simulink model "double_3D_pend_Quat"  (R2023a)
settings: Solver=VariableStepAuto  StartTime=0.0  StopTime=5  MaxStep=1e-3  RelTol=1e-9  AbsTol=1e-9  EnableMultiTasking=on
InitFcn:
  | addpath MuscleForces\
  | addpath EquationsOfMotion\
  | data;
values from neighbouring files (symbols this model uses):
  activation = rand(6,1)    [data.m]    (also in initFunction.m = [0.1,0.5,0.1,0.1,0.1,0.1])
  force = rand(1,6)*500-250    [data.m]
  g = 9.81    [data.m]
  IL = [8.1667, 8.1667, 1.66667,0,0,0]    [data.m]
  IU = [8.1667, 8.1667, 1.66667,0,0,0]    [data.m]
  Ixx = 8.1667    [data.m]
  Iyy = 8.1667    [data.m]
  Izz = 1.66667    [data.m]
  l = 10    [data.m]
  l0m = [20,30,30,30,30,30]    [data.m]
  m = 5    [data.m]
  q1init = q1init/norm(q1init)    [data.m]    (also in initFunction.m)
undefined symbols (not defined in the file or in its folder): initialConditions, X, Y, Z
libraries: sm_lib x33, nesl_utility x15
settings Model: Creator=zoufi  LastModifiedBy=zoufi
settings SolverCC: AutoScaleAbsTol=off  AlgebraicLoopSolver=TrustRegion  MaxZcPerStep=1
settings DataIOCC: LimitDataPoints=on  MaxDataPoints=10000
settings OptimizationCC: ReuseModelBlockBuffer=off  LifeSpan=inf
settings DebuggingCC: UnconnectedInputMsg=warning  UnconnectedOutputMsg=warning  UnconnectedLineMsg=warning  AllowSymbolicDim=off  SubsystemReferenceDiagnosticForUnitTest=warning  SFUnexpectedBacktrackingDiag=warning  SFNoUnconditionalDefaultTransitionDiag=warning  SFExecutionAtInitializationDiag=none  ArithmeticOperatorsInVariantConditions=warning
settings ModelReferenceCC: EnableRefExpFcnMdlSchedulingChecks=on
settings SFSimCC: SimUseLocalCustomCode=off  CustomCodeUndefinedFunction=UseInterfaceOnly
settings RTWCC: RTWUseLocalCustomCode=off  DLArmComputeVersion=19.05
settings CodeAppCC: StateflowObjectComments=on
settings GRTTargetCC: TargetLangStandard=C89/C90 (ANSI)
settings ConfigComp: CovMetricSettings=dw  CovSaveCumulativeToWorkspaceVar=on  CovSaveSingleToWorkspaceVar=on  CovExternalEMLEnable=off  CovSFcnEnable=off
settings SimscapeCC: SimscapeLogType=all  SimscapeLogSimulationStatistics=on  SimscapeLogDataHistory=10000

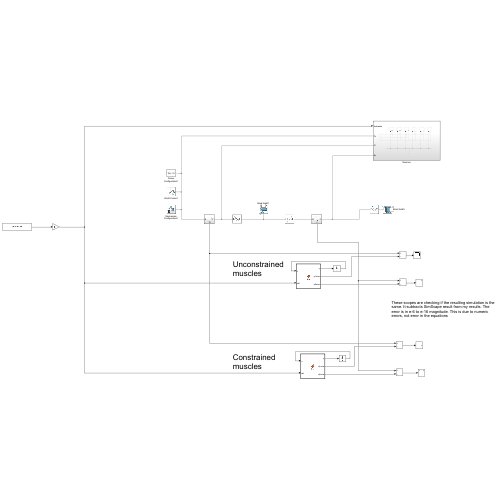
[thumbnail: Simulink's stored preview of the top-level diagram]
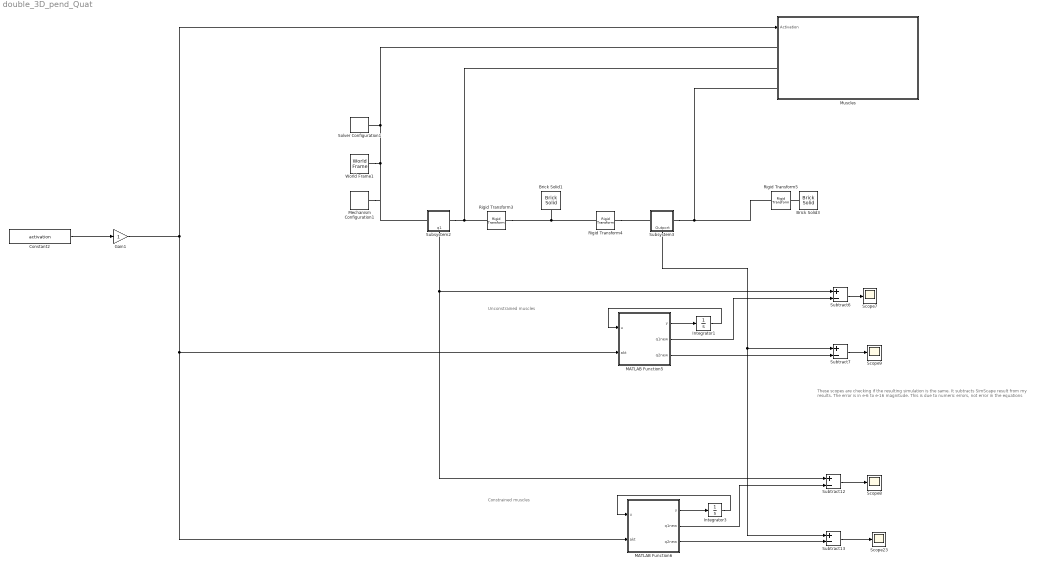
== system double_3D_pend_Quat ==
  note: These scopes are checking if the resulting simulation is the same. It subtracts SimScape result from my results. The error is in e-6 to e-16 magnitude. This is due to numeric errors, not error in the equations
  note: Unconstrained muscles
  note: Constrained muscles
  Brick Solid1 : sm_lib/Body Elements/Brick Solid  GraphicAmbientColor=[0.15 0.15 0.15 1.0]  BasedOnType=Density  BrickDimensions=[1 1 10]  BrickDimensionsUnits=m  CenterOfMass=[0 0 0]  CenterOfMassUnits=m  GraphicDiffuseColor=[0.5 0.5 0.5]  Density=1  DensityUnits=kg/m^3  DoExposeReferenceFrame=on  GraphicEmissiveColor=[0.0 0.0 0.0 1.0]  ExportEntireGeometry=off  SerializedFrames=<Frames><Frame><Id>Frame1</Id><Value><Name>nahore</Name><Origin><Source>GeometricFeature</Source><FeatureName>+z surface</FeatureName></Origin><PrimaryAxis><DefinedDirection>+Z</DefinedDirection><Source>ReferenceFrame</Source><SourceDirection>+Z</SourceDirection><FeatureName></FeatureName></PrimaryAxis><SecondaryAxis><DefinedDirection>+X</DefinedDirection><Source>ReferenceFrame</Source><SourceDirection>+X</SourceDirection><FeatureName></FeatureName></SecondaryAxis></Value></Frame><Frame><Id>Frame2</Id><Value><Name>dole</Name><Origin><Source>GeometricFeature</Source><FeatureName>-z surface</FeatureName></Origin><PrimaryAxis><DefinedDirection>+Z</DefinedDirection><Source>ReferenceFrame</Source><SourceDirection>+Z</SourceDirection><FeatureName></FeatureName></PrimaryAxis><SecondaryAxis><DefinedDirection>+X</DefinedDirection><Source>ReferenceFrame</Source><SourceDirection>+X</SourceDirection><FeatureName></FeatureName></SecondaryAxis></Value></Frame></Frames>  MarkerShape=Sphere  MarkerSize=10  GraphicType=FromGeometry  InertiaType=Custom  Mass=m  MassUnits=kg  MomentsOfInertia=IU(1:3)  MomentsOfInertiaUnits=kg*m^2  GraphicOpacity=1.0  ProductsOfInertia=IU(4:6)  ProductsOfInertiaUnits=kg*m^2  GraphicShininess=75  GraphicSpecularColor=[0.5 0.5 0.5 1.0]  GraphicVisPropType=SimpleVisualProperties
  Brick Solid3 : sm_lib/Body Elements/Brick Solid  GraphicAmbientColor=[0.15 0.15 0.15 1.0]  BasedOnType=Density  BrickDimensions=[1 1 10]  BrickDimensionsUnits=m  CenterOfMass=[0 0 0]  CenterOfMassUnits=m  GraphicDiffuseColor=[0.5 0.5 0.5]  Density=1  DensityUnits=kg/m^3  DoExposeReferenceFrame=on  GraphicEmissiveColor=[0.0 0.0 0.0 1.0]  ExportEntireGeometry=off  SerializedFrames=<Frames><Frame><Id>Frame1</Id><Value><Name>nahore</Name><Origin><Source>GeometricFeature</Source><FeatureName>+z surface</FeatureName></Origin><PrimaryAxis><DefinedDirection>+Z</DefinedDirection><Source>ReferenceFrame</Source><SourceDirection>+Z</SourceDirection><FeatureName></FeatureName></PrimaryAxis><SecondaryAxis><DefinedDirection>+X</DefinedDirection><Source>ReferenceFrame</Source><SourceDirection>+X</SourceDirection><FeatureName></FeatureName></SecondaryAxis></Value></Frame><Frame><Id>Frame2</Id><Value><Name>dole</Name><Origin><Source>GeometricFeature</Source><FeatureName>-z surface</FeatureName></Origin><PrimaryAxis><DefinedDirection>+Z</DefinedDirection><Source>ReferenceFrame</Source><SourceDirection>+Z</SourceDirection><FeatureName></FeatureName></PrimaryAxis><SecondaryAxis><DefinedDirection>+X</DefinedDirection><Source>ReferenceFrame</Source><SourceDirection>+X</SourceDirection><FeatureName></FeatureName></SecondaryAxis></Value></Frame></Frames>  MarkerShape=Sphere  MarkerSize=10  GraphicType=FromGeometry  InertiaType=Custom  Mass=m  MassUnits=kg  MomentsOfInertia=IL(1:3)  MomentsOfInertiaUnits=kg*m^2  GraphicOpacity=1.0  ProductsOfInertia=IL(4:6)  ProductsOfInertiaUnits=kg*m^2  GraphicShininess=75  GraphicSpecularColor=[0.5 0.5 0.5 1.0]  GraphicVisPropType=SimpleVisualProperties
  Constant2 : Constant  Value=activation
  Gain1 : Gain
  Integrator1 : Integrator  InitialCondition=[q1init';q2init';zeros(6,1)]
  Integrator3 : Integrator  InitialCondition=[q1init';q2init';zeros(6,1)]
  MATLAB Function5 : MATLAB Function  TreatAsAtomicUnit=on
  MATLAB Function6 : MATLAB Function  TreatAsAtomicUnit=on
  Mechanism Configuration1 : sm_lib/Utilities/Mechanism Configuration  UniformGravity=Constant  GravityVector=[0 0 -g]  GravityVectorUnits=m/s^2  LinearizationDelta=0.001  JointModeTransitionNonlinearIterations=2
  Muscles : Subsystem
  Rigid Transform3 : sm_lib/Frames and Transforms/Rigid Transform  TranslationMethod=Cartesian  TranslationStandardOffset=0  TranslationStandardOffsetUnits=m  TranslationStandardAxis=+Z  TranslationCartesianOffset=rigid1C  TranslationCartesianOffsetUnits=m  TranslationROffset=0  TranslationROffsetUnits=m  TranslationZOffset=0  TranslationZOffsetUnits=m  TranslationThetaOffset=0  TranslationThetaOffsetUnits=deg  RotationMethod=None  RotationAngleUnits=deg  RotationStandardAxis=+Z  RotationAngle=0.0  RotationArbitraryAxis=[0 0 1]  FollAlignAxisA=+X  BaseAlignAxisA=+Y  FollAlignAxisB=+Y  BaseAlignAxisB=+Z  RotationSequenceAxes=FollowerAxes  RotationSequence=XYX  RotationSequenceAngles=[0 0 0]  RotationSequenceAnglesUnits=deg  RotationMatrix=[1 0 0; 0 1 0; 0 0 1]  Quaternion=[1 0 0 0]
  Rigid Transform4 : sm_lib/Frames and Transforms/Rigid Transform  TranslationMethod=Cartesian  TranslationStandardOffset=0  TranslationStandardOffsetUnits=m  TranslationStandardAxis=+Z  TranslationCartesianOffset=rigid1P  TranslationCartesianOffsetUnits=m  TranslationROffset=0  TranslationROffsetUnits=m  TranslationZOffset=0  TranslationZOffsetUnits=m  TranslationThetaOffset=0  TranslationThetaOffsetUnits=deg  RotationMethod=None  RotationAngleUnits=deg  RotationStandardAxis=+Z  RotationAngle=0.0  RotationArbitraryAxis=[0 0 1]  FollAlignAxisA=+X  BaseAlignAxisA=+Y  FollAlignAxisB=+Y  BaseAlignAxisB=+Z  RotationSequenceAxes=FollowerAxes  RotationSequence=XYX  RotationSequenceAngles=[0 0 0]  RotationSequenceAnglesUnits=deg  RotationMatrix=[1 0 0; 0 1 0; 0 0 1]  Quaternion=[1 0 0 0]
  Rigid Transform5 : sm_lib/Frames and Transforms/Rigid Transform  TranslationMethod=Cartesian  TranslationStandardOffset=0  TranslationStandardOffsetUnits=m  TranslationStandardAxis=+Z  TranslationCartesianOffset=rigid2C  TranslationCartesianOffsetUnits=m  TranslationROffset=0  TranslationROffsetUnits=m  TranslationZOffset=0  TranslationZOffsetUnits=m  TranslationThetaOffset=0  TranslationThetaOffsetUnits=deg  RotationMethod=None  RotationAngleUnits=deg  RotationStandardAxis=+Z  RotationAngle=0.0  RotationArbitraryAxis=[0 0 1]  FollAlignAxisA=+X  BaseAlignAxisA=+Y  FollAlignAxisB=+Y  BaseAlignAxisB=+Z  RotationSequenceAxes=FollowerAxes  RotationSequence=XYX  RotationSequenceAngles=[0 0 0]  RotationSequenceAnglesUnits=deg  RotationMatrix=[1 0 0; 0 1 0; 0 0 1]  Quaternion=[1 0 0 0]
  Scope{7..9,23} (4 alike) : Scope
  Solver Configuration1 : nesl_utility/Solver Configuration  PhysicalDomain=network_engine_domain  SubClassName=solver  LeftPortType=input  RightPortType=generic  Tones=[]  Harmonics=[]  SimulateNoise=off  Profile=off  UseLocalSampling=off  EnableSwitchedLinearOptims=on  FrequencyDomain=off  UseCCode=off  RelTol=0.001  AbsTol=1e-06  MinStep=1e-09  ToWorkspace=off  RevertToSquareIcSolve=off  NumHomotopyIterations=100  PhasorMode=off  PhasorModeNumHarmonics=1  ConsistencySolver=NEWTON_XTOL_AFTER_FTOL  IndexReductionMethod=DerivativeReplacement  DoDC=off  ResidualTolerance=1e-09  ConsistencyTolSource=GLOBAL  ConsistencyAbsTol=0.001  ConsistencyRelTol=0.001  ConsistencyTolFactor=0.001  UseLocalSolver=off  LocalSolverChoice=NE_BACKWARD_EULER_ADVANCER  ResolveIndetEquations=on  FunctionEvalNumThread=1  LocalSolverSampleTime=0.001  DoFixedCost=off  MaxNonlinIter=3  MaxModeIter=2  ComputeImpulses=off  ImpulseIterations=2  LinearAlgebra=Sparse  LinearAlgebraNumThread=0  EquationFormulation=NE_TIME_EF  DelaysMemoryBudget=1024  AutomaticFiltering=on  FilteringTimeConstant=0.001  PartitionStorageMethod=AS_NEEDED  PartitionMemoryBudget=1024  PartitionMethod=FAST
  Subsystem2 : Subsystem
      settings: PortSchema="{\"entries\":[{\"content\":{\"sides\":[{\"content\":{\"connectorIds\":[\"LConn1\"]},\"type\":\"ConnectorPlacement.EquallySpacedRectSide\",\"uuid\":\"8abbfcc9-01b5-41c4-a283-6804113387f6\"},{\"content\":{\"connectorIds\":[\"RConn1\"],\"side\":\"RIGHT\"},\"type\":\"ConnectorPlacement.EquallySpacedRectSide\",\"uuid\":\"0343473e-44e7-4112-89d1-12c32e7e714a\"},{\"content\":{\"side\":\"TOP\"},\"type\":\"ConnectorPlacement.EquallySpacedRectSide\",\"uuid\":\"e3f3e934-10bc-4ce8-a108-92e62f8cce45\"},{\"content\":{\"connectorIds\":[\"Out1\"],\"side\":\"BOTTOM\"},\"type\":\"ConnectorPlacement.EquallySpacedRectSide\",\"uuid\":\"88cd244a-d5e6-4fc3-9229-ab44331ab4a2\"}]},\"type\":\"ConnectorPlacement.EquallySpacedConnector\",\"uuid\":\"3b604a58-c197-4bd4-84dd-7dfe8ba758a8\"}],\"packageUris\":[\"http://schema.mathworks.com/mf0/Connector/R2020b\"],\"version\":\"1.0\"}"
  Subsystem3 : Subsystem
      settings: PortSchema="{\"entries\":[{\"content\":{\"sides\":[{\"content\":{\"connectorIds\":[\"LConn1\"]},\"type\":\"ConnectorPlacement.EquallySpacedRectSide\",\"uuid\":\"a7767b74-3ef3-4a0a-9db8-74df01f0c76b\"},{\"content\":{\"connectorIds\":[\"RConn1\"],\"side\":\"RIGHT\"},\"type\":\"ConnectorPlacement.EquallySpacedRectSide\",\"uuid\":\"2f8f74c3-a8e5-4e43-9dec-7e8e5a722b87\"},{\"content\":{\"side\":\"TOP\"},\"type\":\"ConnectorPlacement.EquallySpacedRectSide\",\"uuid\":\"fe0d2add-2cc5-4054-90cf-1ce1d94f501e\"},{\"content\":{\"connectorIds\":[\"Out1\"],\"side\":\"BOTTOM\"},\"type\":\"ConnectorPlacement.EquallySpacedRectSide\",\"uuid\":\"7824871f-3418-47cc-a708-554774ed2fda\"}]},\"type\":\"ConnectorPlacement.EquallySpacedConnector\",\"uuid\":\"6ea328c6-953a-4acc-92cd-0e7443fdf9ea\"}],\"packageUris\":[\"http://schema.mathworks.com/mf0/Connector/R2020b\"],\"version\":\"1.0\"}"
  Subtract{6..7,12..13} (4 alike) : Sum  Inputs=+-
  World Frame1 : sm_lib/Frames and Transforms/World Frame
  wires:
  Constant2/1 -> Gain1/1
  MATLAB Function5/1(y) -> Integrator1/1
  Integrator1/1 -> MATLAB Function5/1(u)
  MATLAB Function5/2(q1new) -> Subtract6/2
  Subtract6/1 -> Scope7/1
  MATLAB Function5/3(q2new) -> Subtract7/2
  Subtract7/1 -> Scope9/1
  Subsystem3/1(Outport) -> Subtract13/1, Subtract7/1
  Subtract13/1 -> Scope23/1
  MATLAB Function6/3(q2new) -> Subtract13/2
  Subtract12/1 -> Scope8/1
  MATLAB Function6/2(q1new) -> Subtract12/2
  Subsystem2/1(q1) -> Subtract12/1, Subtract6/1
  Integrator3/1 -> MATLAB Function6/1(u)
  MATLAB Function6/1(y) -> Integrator3/1
  Gain1/1 -> Muscles/1(Activation), MATLAB Function6/2(akt), MATLAB Function5/2(akt)
  connections:
  World Frame1/RConn1 -- Muscles/LConn1 -- Solver Configuration1/RConn1 -- Subsystem2/LConn1 -- Mechanism Configuration1/RConn1
  Subsystem2/RConn1 -- Muscles/LConn2 -- Rigid Transform3/RConn1
  Rigid Transform3/LConn1 -- Rigid Transform4/LConn1 -- Brick Solid1/RConn1
  Brick Solid3/RConn1 -- Rigid Transform5/LConn1
  Subsystem3/RConn1 -- Muscles/LConn3 -- Rigid Transform5/RConn1
  Rigid Transform4/RConn1 -- Subsystem3/LConn1

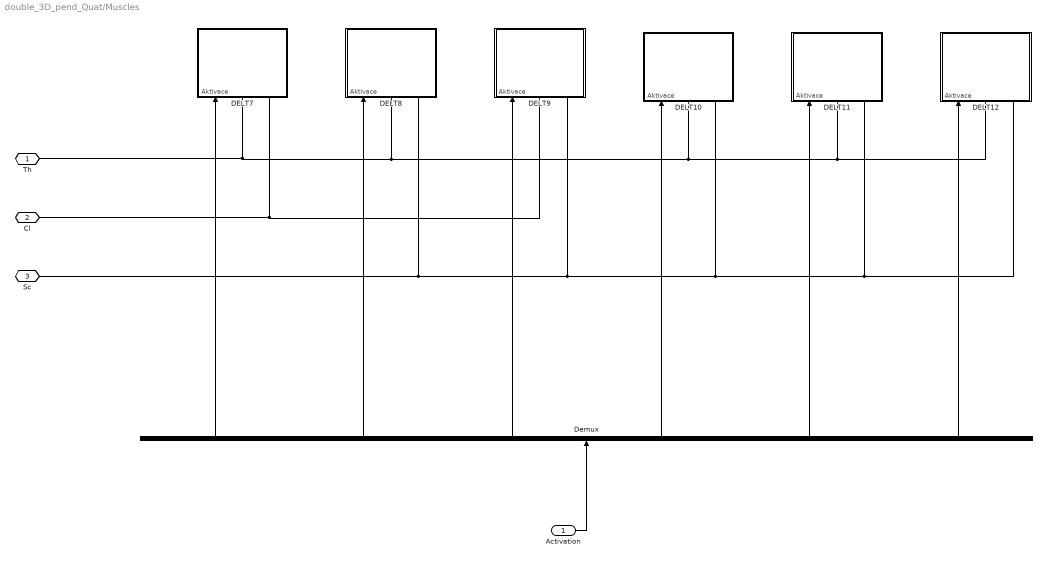
== system double_3D_pend_Quat/Muscles ==
  Activation : Inport
  DELT10 : Subsystem
  DELT11 : Subsystem
  DELT12 : Subsystem
  DELT7 : Subsystem
  DELT8 : Subsystem
  DELT9 : Subsystem
  Demux : Demux  Outputs=6
  Th : PMIOPort  Side=Left
  Cl : PMIOPort  Port=2  Side=Left
  Sc : PMIOPort  Port=3  Side=Left
  wires:
  Demux/1 -> DELT7/1(Aktivace)
  Demux/2 -> DELT8/1(Aktivace)
  Demux/3 -> DELT9/1(Aktivace)
  Demux/4 -> DELT10/1(Aktivace)
  Demux/5 -> DELT11/1(Aktivace)
  Demux/6 -> DELT12/1(Aktivace)
  Activation/1 -> Demux/1
  connections:
  DELT7/LConn1 -- DELT12/LConn1 -- DELT11/LConn1 -- DELT10/LConn1 -- DELT8/LConn1 -- Th/RConn1
  DELT7/LConn2 -- DELT9/LConn1 -- Cl/RConn1
  DELT8/LConn2 -- DELT12/LConn2 -- DELT11/LConn2 -- DELT10/LConn2 -- DELT9/LConn2 -- Sc/RConn1

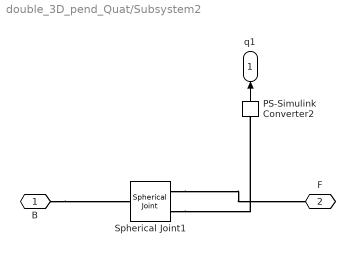
== system double_3D_pend_Quat/Subsystem2 ==
  PS-Simulink Converter2 : nesl_utility/PS-Simulink Converter  PhysicalDomain=network_engine_domain  SubClassName=ps_output  LeftPortType=input  RightPortType=output  PseudoPeriodic=off  Frequencies=[]  VectorFormat=inherit  Unit=inherit  AffineConversion=off
  Spherical Joint1 : sm_lib/Joints/Spherical Joint  JointMode=Normal  SenseConstraintForce=off  SenseConstraintForceX=off  SenseConstraintForceY=off  SenseConstraintForceZ=off  SenseConstraintTorque=off  SenseConstraintTorqueX=off  SenseConstraintTorqueY=off  SenseConstraintTorqueZ=off  SenseTotalForce=off  SenseTotalForceX=off  SenseTotalForceY=off  SenseTotalForceZ=off  SenseTotalTorque=off  SenseTotalTorqueX=off  SenseTotalTorqueY=off  SenseTotalTorqueZ=off  CompositeWrenchDir=BaseOnFollower  CompositeWrenchFrame=BaseFrame  EqPosRotationMethod=None  EqPosRotationAngleUnits=deg  EqPosRotationStandardAxis=+Z  EqPosRotationAngle=0.0  EqPosRotationArbitraryAxis=[0 0 1]  EqPosFollAlignAxisA=+X  EqPosBaseAlignAxisA=+Y  EqPosFollAlignAxisB=+Y  EqPosBaseAlignAxisB=+Z  EqPosRotationSequenceAxes=FollowerAxes  EqPosRotationSequence=XYX  EqPosRotationSequenceAngles=[0 0 0]  EqPosRotationSequenceAnglesUnits=deg  EqPosRotationMatrix=[1 0 0; 0 1 0; 0 0 1]  EqPosQuaternion=[1 0 0 0]  SpringStiffness=0  SpringStiffnessUnits=N*m/deg  DampingCoefficient=c  DampingCoefficientUnits=N*m/(rad/s)  ActuateTorqueX=off  ActuateTorqueY=off  ActuateTorqueZ=off  ActuateTorque=off  TorqueActuationMode=InputTorque  MotionActuationMode=ComputedMotion  ActuationFrame=FollowerFrame  SensePosition=on  SenseVelocityX=off  SenseVelocityY=off  SenseVelocityZ=off  SenseVelocity=off  SenseAccelerationX=off  SenseAccelerationY=off  SenseAccelerationZ=off  SenseAcceleration=off  SenseTorqueX=off  SenseTorqueY=off  SenseTorqueZ=off  SenseTorqueForce=off  SenseLowerLimitTorqueMag=off  SenseUpperLimitTorqueMag=off  SensingFrame=BaseFrame  LowerLimitSpecify=off  LowerLimitBound=15  LowerLimitBoundUnits=deg  LowerLimitStiffness=1e4  LowerLimitStiffnessUnits=N*m/deg  LowerLimitDamping=10  LowerLimitDampingUnits=N*m/(deg/s)  LowerLimitTransitionRegionWidth=0.1  LowerLimitTransitionRegionWidthUnits=deg  UpperLimitSpecify=off  UpperLimitBound=45  UpperLimitBoundUnits=deg  UpperLimitStiffness=1e4  UpperLimitStiffnessUnits=N*m/deg  UpperLimitDamping=10  UpperLimitDampingUnits=N*m/(deg/s)  UpperLimitTransitionRegionWidth=0.1  UpperLimitTransitionRegionWidthUnits=deg  PositionTargetRotationMethod=Quaternion  PositionTargetRotationAngleUnits=deg  PositionTargetRotationStandardAxis=+Z  PositionTargetRotationAngle=0.0  PositionTargetRotationArbitraryAxis=[0 0 1]  PositionTargetFollAlignAxisA=+X  PositionTargetBaseAlignAxisA=+Y  PositionTargetFollAlignAxisB=+Y  PositionTargetBaseAlignAxisB=+Z  PositionTargetRotationSequenceAxes=FollowerAxes  PositionTargetRotationSequence=XYZ  PositionTargetRotationSequenceAngles=initialConditions(1:3)  PositionTargetRotationSequenceAnglesUnits=rad  PositionTargetRotationMatrix=[1 0 0; 0 1 0; 0 0 1]  PositionTargetQuaternion=q1init  PositionTargetSpecify=on  PositionTargetPriority=High  VelocityTargetValue=[0 0 0]  VelocityTargetValueUnits=deg/s  VelocityTargetSpecify=off  VelocityTargetPriority=High  VelocityTargetInFollowerFrame=on
  B : PMIOPort  Side=Left
  F : PMIOPort  Port=2  Side=Right
  q1 : Outport
  wires:
  PS-Simulink Converter2/1 -> q1/1
  connections:
  Spherical Joint1/RConn2 -- PS-Simulink Converter2/LConn1
  Spherical Joint1/RConn1 -- F/RConn1
  B/RConn1 -- Spherical Joint1/LConn1

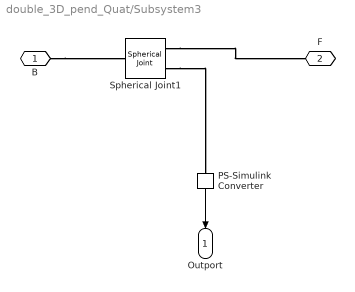
== system double_3D_pend_Quat/Subsystem3 ==
  PS-Simulink Converter : nesl_utility/PS-Simulink Converter  PhysicalDomain=network_engine_domain  SubClassName=ps_output  LeftPortType=input  RightPortType=output  PseudoPeriodic=off  Frequencies=[]  VectorFormat=inherit  Unit=inherit  AffineConversion=off
  Spherical Joint1 : sm_lib/Joints/Spherical Joint  JointMode=Normal  SenseConstraintForce=off  SenseConstraintForceX=off  SenseConstraintForceY=off  SenseConstraintForceZ=off  SenseConstraintTorque=off  SenseConstraintTorqueX=off  SenseConstraintTorqueY=off  SenseConstraintTorqueZ=off  SenseTotalForce=off  SenseTotalForceX=off  SenseTotalForceY=off  SenseTotalForceZ=off  SenseTotalTorque=off  SenseTotalTorqueX=off  SenseTotalTorqueY=off  SenseTotalTorqueZ=off  CompositeWrenchDir=FollowerOnBase  CompositeWrenchFrame=BaseFrame  EqPosRotationMethod=None  EqPosRotationAngleUnits=deg  EqPosRotationStandardAxis=+Z  EqPosRotationAngle=0.0  EqPosRotationArbitraryAxis=[0 0 1]  EqPosFollAlignAxisA=+X  EqPosBaseAlignAxisA=+Y  EqPosFollAlignAxisB=+Y  EqPosBaseAlignAxisB=+Z  EqPosRotationSequenceAxes=FollowerAxes  EqPosRotationSequence=XYX  EqPosRotationSequenceAngles=[0 0 0]  EqPosRotationSequenceAnglesUnits=deg  EqPosRotationMatrix=[1 0 0; 0 1 0; 0 0 1]  EqPosQuaternion=[1 0 0 0]  SpringStiffness=0  SpringStiffnessUnits=N*m/deg  DampingCoefficient=c  DampingCoefficientUnits=N*m/(rad/s)  ActuateTorqueX=off  ActuateTorqueY=off  ActuateTorqueZ=off  ActuateTorque=off  TorqueActuationMode=InputTorque  MotionActuationMode=ComputedMotion  ActuationFrame=FollowerFrame  SensePosition=on  SenseVelocityX=off  SenseVelocityY=off  SenseVelocityZ=off  SenseVelocity=off  SenseAccelerationX=off  SenseAccelerationY=off  SenseAccelerationZ=off  SenseAcceleration=off  SenseTorqueX=off  SenseTorqueY=off  SenseTorqueZ=off  SenseTorqueForce=off  SenseLowerLimitTorqueMag=off  SenseUpperLimitTorqueMag=off  SensingFrame=BaseFrame  LowerLimitSpecify=off  LowerLimitBound=15  LowerLimitBoundUnits=deg  LowerLimitStiffness=1e4  LowerLimitStiffnessUnits=N*m/deg  LowerLimitDamping=10  LowerLimitDampingUnits=N*m/(deg/s)  LowerLimitTransitionRegionWidth=0.1  LowerLimitTransitionRegionWidthUnits=deg  UpperLimitSpecify=off  UpperLimitBound=45  UpperLimitBoundUnits=deg  UpperLimitStiffness=1e4  UpperLimitStiffnessUnits=N*m/deg  UpperLimitDamping=10  UpperLimitDampingUnits=N*m/(deg/s)  UpperLimitTransitionRegionWidth=0.1  UpperLimitTransitionRegionWidthUnits=deg  PositionTargetRotationMethod=Quaternion  PositionTargetRotationAngleUnits=deg  PositionTargetRotationStandardAxis=+Z  PositionTargetRotationAngle=0.0  PositionTargetRotationArbitraryAxis=[0 0 1]  PositionTargetFollAlignAxisA=+X  PositionTargetBaseAlignAxisA=+Y  PositionTargetFollAlignAxisB=+Y  PositionTargetBaseAlignAxisB=+Z  PositionTargetRotationSequenceAxes=FollowerAxes  PositionTargetRotationSequence=XYZ  PositionTargetRotationSequenceAngles=initialConditions(4:6)  PositionTargetRotationSequenceAnglesUnits=rad  PositionTargetRotationMatrix=[1 0 0; 0 1 0; 0 0 1]  PositionTargetQuaternion=q2init  PositionTargetSpecify=on  PositionTargetPriority=High  VelocityTargetValue=[0 0 0]  VelocityTargetValueUnits=deg/s  VelocityTargetSpecify=off  VelocityTargetPriority=High  VelocityTargetInFollowerFrame=on
  B : PMIOPort  Side=Left
  F : PMIOPort  Port=2  Side=Right
  Outport : Outport
  wires:
  PS-Simulink Converter/1 -> Outport/1
  connections:
  B/RConn1 -- Spherical Joint1/LConn1
  Spherical Joint1/RConn1 -- F/RConn1
  Spherical Joint1/RConn2 -- PS-Simulink Converter/LConn1

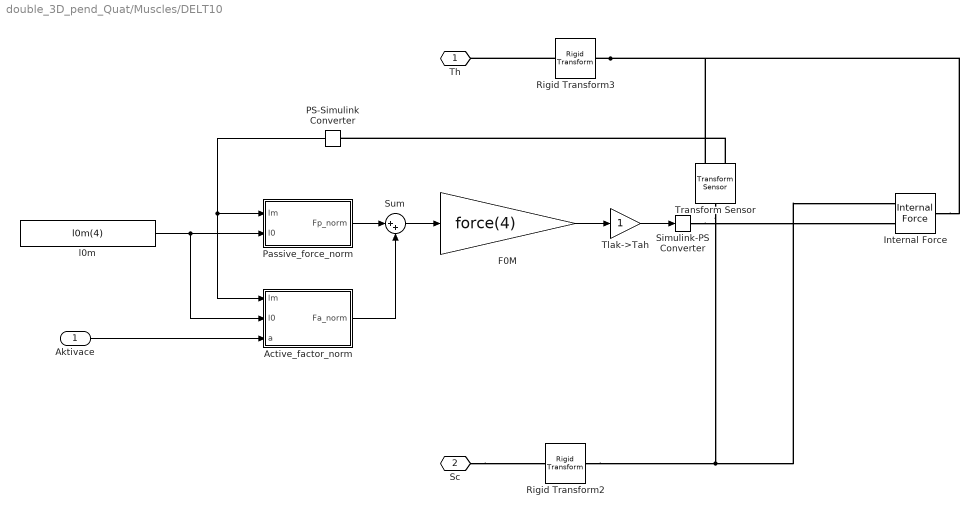
== system double_3D_pend_Quat/Muscles/DELT10 ==
  Aktivace : Inport
  Active_factor_norm : MATLAB Function  TreatAsAtomicUnit=on
  F0M : Gain  Gain=force(4)
  Internal Force : sm_lib/Forces and Torques/Internal Force
  PS-Simulink Converter : nesl_utility/PS-Simulink Converter  PhysicalDomain=network_engine_domain  SubClassName=ps_output  LeftPortType=input  RightPortType=output  PseudoPeriodic=off  Frequencies=[]  VectorFormat=inherit  Unit=inherit  AffineConversion=off
  Passive_force_norm : MATLAB Function  TreatAsAtomicUnit=on
  Rigid Transform2 : sm_lib/Frames and Transforms/Rigid Transform  TranslationMethod=Cartesian  TranslationStandardOffset=0  TranslationStandardOffsetUnits=m  TranslationStandardAxis=+Z  TranslationCartesianOffset=[2,-2,5]  TranslationCartesianOffsetUnits=m  TranslationROffset=0  TranslationROffsetUnits=m  TranslationZOffset=0  TranslationZOffsetUnits=m  TranslationThetaOffset=0  TranslationThetaOffsetUnits=deg  RotationMethod=None  RotationAngleUnits=deg  RotationStandardAxis=+Z  RotationAngle=0.0  RotationArbitraryAxis=[0 0 1]  FollAlignAxisA=+X  BaseAlignAxisA=+Y  FollAlignAxisB=+Y  BaseAlignAxisB=+Z  RotationSequenceAxes=FollowerAxes  RotationSequence=XYX  RotationSequenceAngles=[0 0 0]  RotationSequenceAnglesUnits=deg  RotationMatrix=[1 0 0; 0 1 0; 0 0 1]  Quaternion=[1 0 0 0]
  Rigid Transform3 : sm_lib/Frames and Transforms/Rigid Transform  TranslationMethod=Cartesian  TranslationStandardOffset=0  TranslationStandardOffsetUnits=m  TranslationStandardAxis=+Z  TranslationCartesianOffset=[-6, -6, 0]  TranslationCartesianOffsetUnits=m  TranslationROffset=0  TranslationROffsetUnits=m  TranslationZOffset=0  TranslationZOffsetUnits=m  TranslationThetaOffset=0  TranslationThetaOffsetUnits=deg  RotationMethod=None  RotationAngleUnits=deg  RotationStandardAxis=+Z  RotationAngle=0.0  RotationArbitraryAxis=[0 0 1]  FollAlignAxisA=+X  BaseAlignAxisA=+Y  FollAlignAxisB=+Y  BaseAlignAxisB=+Z  RotationSequenceAxes=FollowerAxes  RotationSequence=XYX  RotationSequenceAngles=[0 0 0]  RotationSequenceAnglesUnits=deg  RotationMatrix=[1 0 0; 0 1 0; 0 0 1]  Quaternion=[1 0 0 0]
  Simulink-PS Converter : nesl_utility/Simulink-PS Converter  PhysicalDomain=network_engine_domain  SubClassName=ps_input  LeftPortType=input  RightPortType=output  PseudoPeriodic=off  Frequencies=[]  NoiseDistribution=none  NoiseParameters=[]  Unit=1  AffineConversion=off  FilteringAndDerivatives=provide  SimscapeFilterOrder=1  InputFilterTimeConstant=0.001  UdotUserProvided=0
  Sum : Sum  Inputs=|++
  Tlak->Tah : Gain
  Transform Sensor : sm_lib/Frames and Transforms/Transform Sensor  MeasurementFrame=World  RotationSequence=XYX  SenseAngle=off  SenseAxis=off  SenseQ=off  SenseR=off  SenseRotationSequence=off  SenseOmegaX=off  SenseOmegaY=off  SenseOmegaZ=off  SenseQDot=off  SenseRDot=off  SenseRotationSequenceDot=off  SenseAlphaX=off  SenseAlphaY=off  SenseAlphaZ=off  SenseQDDot=off  SenseRDDot=off  SenseX=off  SenseY=off  SenseZ=off  SenseRad=off  SenseAzim=off  SenseDist=on  SenseInc=off  SenseXDot=off  SenseYDot=off  SenseZDot=off  SenseRadDot=off  SenseAzimDot=off  SenseDistDot=off  SenseIncDot=off  SenseXDDot=off  SenseYDDot=off  SenseZDDot=off  SenseRadDDot=off  SenseAzimDDot=off  SenseDistDDot=off  SenseIncDDot=off
  l0m : Constant  Value=l0m(4)
  Th : PMIOPort  Side=Left
  Sc : PMIOPort  Port=2  Side=Left
  wires:
  Aktivace/1 -> Active_factor_norm/3(a)
  l0m/1 -> Passive_force_norm/2(l0), Active_factor_norm/2(l0)
  PS-Simulink Converter/1 -> Passive_force_norm/1(lm), Active_factor_norm/1(lm)
  Tlak->Tah/1 -> Simulink-PS Converter/1
  Active_factor_norm/1(Fa_norm) -> Sum/2
  Passive_force_norm/1(Fp_norm) -> Sum/1
  F0M/1 -> Tlak->Tah/1
  Sum/1 -> F0M/1
  connections:
  Transform Sensor/RConn2 -- PS-Simulink Converter/LConn1
  Simulink-PS Converter/RConn1 -- Internal Force/LConn2
  Rigid Transform3/RConn1 -- Transform Sensor/RConn1 -- Internal Force/RConn1
  Transform Sensor/LConn1 -- Rigid Transform2/RConn1 -- Internal Force/LConn1
  Rigid Transform3/LConn1 -- Th/RConn1
  Sc/RConn1 -- Rigid Transform2/LConn1

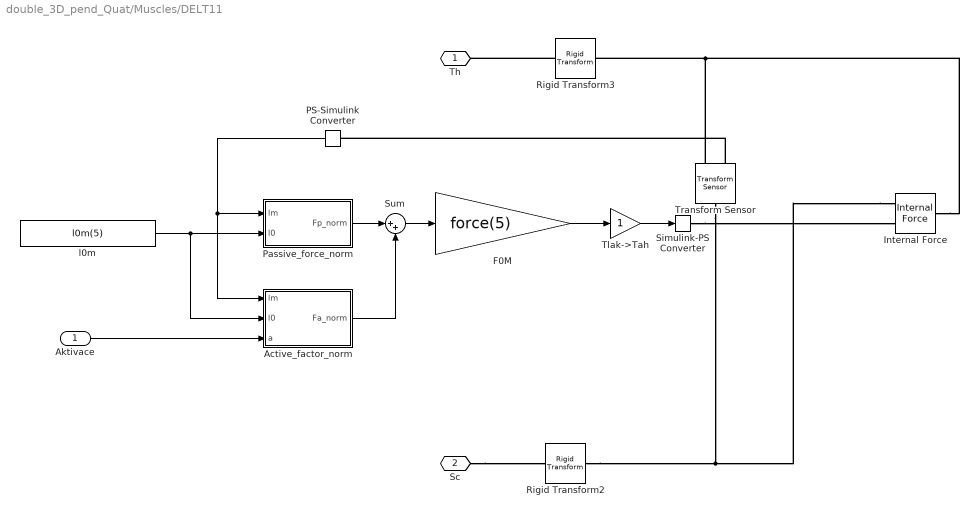
== system double_3D_pend_Quat/Muscles/DELT11 ==
  Aktivace : Inport
  Active_factor_norm : MATLAB Function  TreatAsAtomicUnit=on
  F0M : Gain  Gain=force(5)
  Internal Force : sm_lib/Forces and Torques/Internal Force
  PS-Simulink Converter : nesl_utility/PS-Simulink Converter  PhysicalDomain=network_engine_domain  SubClassName=ps_output  LeftPortType=input  RightPortType=output  PseudoPeriodic=off  Frequencies=[]  VectorFormat=inherit  Unit=inherit  AffineConversion=off
  Passive_force_norm : MATLAB Function  TreatAsAtomicUnit=on
  Rigid Transform2 : sm_lib/Frames and Transforms/Rigid Transform  TranslationMethod=Cartesian  TranslationStandardOffset=0  TranslationStandardOffsetUnits=m  TranslationStandardAxis=+Z  TranslationCartesianOffset=[-3,-3,0]  TranslationCartesianOffsetUnits=m  TranslationROffset=0  TranslationROffsetUnits=m  TranslationZOffset=0  TranslationZOffsetUnits=m  TranslationThetaOffset=0  TranslationThetaOffsetUnits=deg  RotationMethod=None  RotationAngleUnits=deg  RotationStandardAxis=+Z  RotationAngle=0.0  RotationArbitraryAxis=[0 0 1]  FollAlignAxisA=+X  BaseAlignAxisA=+Y  FollAlignAxisB=+Y  BaseAlignAxisB=+Z  RotationSequenceAxes=FollowerAxes  RotationSequence=XYX  RotationSequenceAngles=[0 0 0]  RotationSequenceAnglesUnits=deg  RotationMatrix=[1 0 0; 0 1 0; 0 0 1]  Quaternion=[1 0 0 0]
  Rigid Transform3 : sm_lib/Frames and Transforms/Rigid Transform  TranslationMethod=Cartesian  TranslationStandardOffset=0  TranslationStandardOffsetUnits=m  TranslationStandardAxis=+Z  TranslationCartesianOffset=[-7, 5, 0]  TranslationCartesianOffsetUnits=m  TranslationROffset=0  TranslationROffsetUnits=m  TranslationZOffset=0  TranslationZOffsetUnits=m  TranslationThetaOffset=0  TranslationThetaOffsetUnits=deg  RotationMethod=None  RotationAngleUnits=deg  RotationStandardAxis=+Z  RotationAngle=0.0  RotationArbitraryAxis=[0 0 1]  FollAlignAxisA=+X  BaseAlignAxisA=+Y  FollAlignAxisB=+Y  BaseAlignAxisB=+Z  RotationSequenceAxes=FollowerAxes  RotationSequence=XYX  RotationSequenceAngles=[0 0 0]  RotationSequenceAnglesUnits=deg  RotationMatrix=[1 0 0; 0 1 0; 0 0 1]  Quaternion=[1 0 0 0]
  Simulink-PS Converter : nesl_utility/Simulink-PS Converter  PhysicalDomain=network_engine_domain  SubClassName=ps_input  LeftPortType=input  RightPortType=output  PseudoPeriodic=off  Frequencies=[]  NoiseDistribution=none  NoiseParameters=[]  Unit=1  AffineConversion=off  FilteringAndDerivatives=provide  SimscapeFilterOrder=1  InputFilterTimeConstant=0.001  UdotUserProvided=0
  Sum : Sum  Inputs=|++
  Tlak->Tah : Gain
  Transform Sensor : sm_lib/Frames and Transforms/Transform Sensor  MeasurementFrame=World  RotationSequence=XYX  SenseAngle=off  SenseAxis=off  SenseQ=off  SenseR=off  SenseRotationSequence=off  SenseOmegaX=off  SenseOmegaY=off  SenseOmegaZ=off  SenseQDot=off  SenseRDot=off  SenseRotationSequenceDot=off  SenseAlphaX=off  SenseAlphaY=off  SenseAlphaZ=off  SenseQDDot=off  SenseRDDot=off  SenseX=off  SenseY=off  SenseZ=off  SenseRad=off  SenseAzim=off  SenseDist=on  SenseInc=off  SenseXDot=off  SenseYDot=off  SenseZDot=off  SenseRadDot=off  SenseAzimDot=off  SenseDistDot=off  SenseIncDot=off  SenseXDDot=off  SenseYDDot=off  SenseZDDot=off  SenseRadDDot=off  SenseAzimDDot=off  SenseDistDDot=off  SenseIncDDot=off
  l0m : Constant  Value=l0m(5)
  Th : PMIOPort  Side=Left
  Sc : PMIOPort  Port=2  Side=Left
  wires:
  Sum/1 -> F0M/1
  F0M/1 -> Tlak->Tah/1
  Passive_force_norm/1(Fp_norm) -> Sum/1
  Active_factor_norm/1(Fa_norm) -> Sum/2
  Tlak->Tah/1 -> Simulink-PS Converter/1
  PS-Simulink Converter/1 -> Active_factor_norm/1(lm), Passive_force_norm/1(lm)
  l0m/1 -> Active_factor_norm/2(l0), Passive_force_norm/2(l0)
  Aktivace/1 -> Active_factor_norm/3(a)
  connections:
  Sc/RConn1 -- Rigid Transform2/LConn1
  Rigid Transform3/LConn1 -- Th/RConn1
  Internal Force/LConn1 -- Rigid Transform2/RConn1 -- Transform Sensor/LConn1
  Internal Force/RConn1 -- Transform Sensor/RConn1 -- Rigid Transform3/RConn1
  Simulink-PS Converter/RConn1 -- Internal Force/LConn2
  Transform Sensor/RConn2 -- PS-Simulink Converter/LConn1

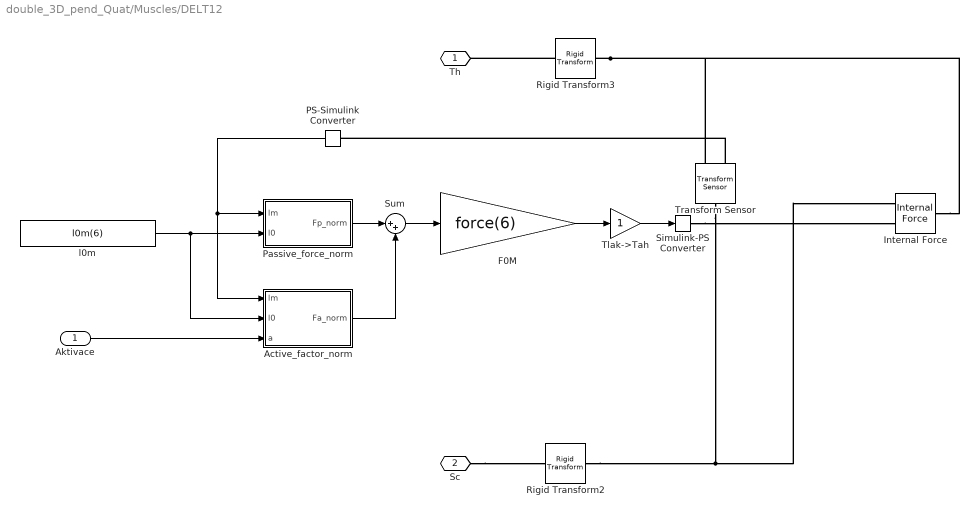
== system double_3D_pend_Quat/Muscles/DELT12 ==
  Aktivace : Inport
  Active_factor_norm : MATLAB Function  TreatAsAtomicUnit=on
  F0M : Gain  Gain=force(6)
  Internal Force : sm_lib/Forces and Torques/Internal Force
  PS-Simulink Converter : nesl_utility/PS-Simulink Converter  PhysicalDomain=network_engine_domain  SubClassName=ps_output  LeftPortType=input  RightPortType=output  PseudoPeriodic=off  Frequencies=[]  VectorFormat=inherit  Unit=inherit  AffineConversion=off
  Passive_force_norm : MATLAB Function  TreatAsAtomicUnit=on
  Rigid Transform2 : sm_lib/Frames and Transforms/Rigid Transform  TranslationMethod=Cartesian  TranslationStandardOffset=0  TranslationStandardOffsetUnits=m  TranslationStandardAxis=+Z  TranslationCartesianOffset=[-4,4,-4]  TranslationCartesianOffsetUnits=m  TranslationROffset=0  TranslationROffsetUnits=m  TranslationZOffset=0  TranslationZOffsetUnits=m  TranslationThetaOffset=0  TranslationThetaOffsetUnits=deg  RotationMethod=None  RotationAngleUnits=deg  RotationStandardAxis=+Z  RotationAngle=0.0  RotationArbitraryAxis=[0 0 1]  FollAlignAxisA=+X  BaseAlignAxisA=+Y  FollAlignAxisB=+Y  BaseAlignAxisB=+Z  RotationSequenceAxes=FollowerAxes  RotationSequence=XYX  RotationSequenceAngles=[0 0 0]  RotationSequenceAnglesUnits=deg  RotationMatrix=[1 0 0; 0 1 0; 0 0 1]  Quaternion=[1 0 0 0]
  Rigid Transform3 : sm_lib/Frames and Transforms/Rigid Transform  TranslationMethod=Cartesian  TranslationStandardOffset=0  TranslationStandardOffsetUnits=m  TranslationStandardAxis=+Z  TranslationCartesianOffset=[8, -4, 0]  TranslationCartesianOffsetUnits=m  TranslationROffset=0  TranslationROffsetUnits=m  TranslationZOffset=0  TranslationZOffsetUnits=m  TranslationThetaOffset=0  TranslationThetaOffsetUnits=deg  RotationMethod=None  RotationAngleUnits=deg  RotationStandardAxis=+Z  RotationAngle=0.0  RotationArbitraryAxis=[0 0 1]  FollAlignAxisA=+X  BaseAlignAxisA=+Y  FollAlignAxisB=+Y  BaseAlignAxisB=+Z  RotationSequenceAxes=FollowerAxes  RotationSequence=XYX  RotationSequenceAngles=[0 0 0]  RotationSequenceAnglesUnits=deg  RotationMatrix=[1 0 0; 0 1 0; 0 0 1]  Quaternion=[1 0 0 0]
  Simulink-PS Converter : nesl_utility/Simulink-PS Converter  PhysicalDomain=network_engine_domain  SubClassName=ps_input  LeftPortType=input  RightPortType=output  PseudoPeriodic=off  Frequencies=[]  NoiseDistribution=none  NoiseParameters=[]  Unit=1  AffineConversion=off  FilteringAndDerivatives=provide  SimscapeFilterOrder=1  InputFilterTimeConstant=0.001  UdotUserProvided=0
  Sum : Sum  Inputs=|++
  Tlak->Tah : Gain
  Transform Sensor : sm_lib/Frames and Transforms/Transform Sensor  MeasurementFrame=World  RotationSequence=XYX  SenseAngle=off  SenseAxis=off  SenseQ=off  SenseR=off  SenseRotationSequence=off  SenseOmegaX=off  SenseOmegaY=off  SenseOmegaZ=off  SenseQDot=off  SenseRDot=off  SenseRotationSequenceDot=off  SenseAlphaX=off  SenseAlphaY=off  SenseAlphaZ=off  SenseQDDot=off  SenseRDDot=off  SenseX=off  SenseY=off  SenseZ=off  SenseRad=off  SenseAzim=off  SenseDist=on  SenseInc=off  SenseXDot=off  SenseYDot=off  SenseZDot=off  SenseRadDot=off  SenseAzimDot=off  SenseDistDot=off  SenseIncDot=off  SenseXDDot=off  SenseYDDot=off  SenseZDDot=off  SenseRadDDot=off  SenseAzimDDot=off  SenseDistDDot=off  SenseIncDDot=off
  l0m : Constant  Value=l0m(6)
  Th : PMIOPort  Side=Left
  Sc : PMIOPort  Port=2  Side=Left
  wires:
  Aktivace/1 -> Active_factor_norm/3(a)
  l0m/1 -> Passive_force_norm/2(l0), Active_factor_norm/2(l0)
  PS-Simulink Converter/1 -> Passive_force_norm/1(lm), Active_factor_norm/1(lm)
  Tlak->Tah/1 -> Simulink-PS Converter/1
  Active_factor_norm/1(Fa_norm) -> Sum/2
  Passive_force_norm/1(Fp_norm) -> Sum/1
  F0M/1 -> Tlak->Tah/1
  Sum/1 -> F0M/1
  connections:
  Transform Sensor/RConn2 -- PS-Simulink Converter/LConn1
  Simulink-PS Converter/RConn1 -- Internal Force/LConn2
  Rigid Transform3/RConn1 -- Transform Sensor/RConn1 -- Internal Force/RConn1
  Transform Sensor/LConn1 -- Rigid Transform2/RConn1 -- Internal Force/LConn1
  Rigid Transform3/LConn1 -- Th/RConn1
  Sc/RConn1 -- Rigid Transform2/LConn1

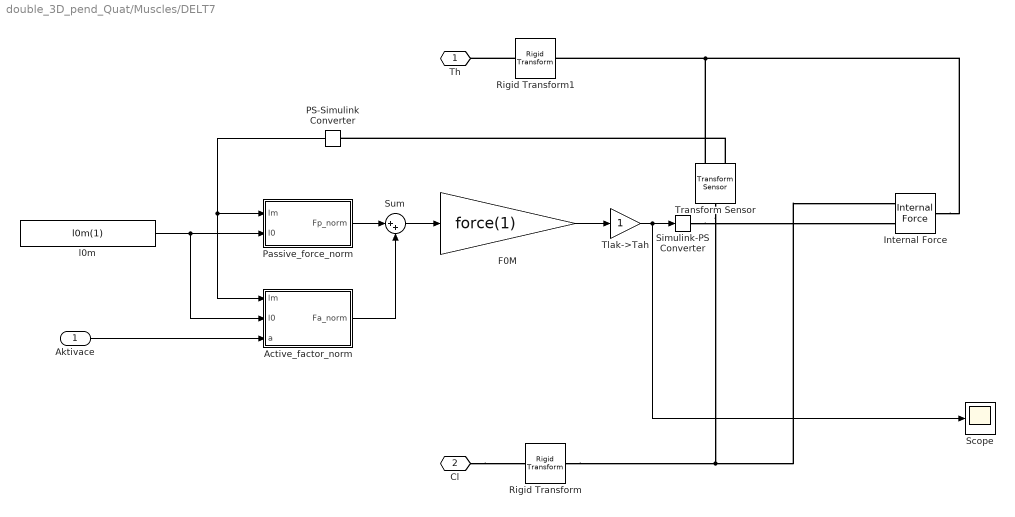
== system double_3D_pend_Quat/Muscles/DELT7 ==
  Aktivace : Inport
  Active_factor_norm : MATLAB Function  TreatAsAtomicUnit=on
  F0M : Gain  Gain=force(1)
  Internal Force : sm_lib/Forces and Torques/Internal Force
  PS-Simulink Converter : nesl_utility/PS-Simulink Converter  PhysicalDomain=network_engine_domain  SubClassName=ps_output  LeftPortType=input  RightPortType=output  PseudoPeriodic=off  Frequencies=[]  VectorFormat=inherit  Unit=inherit  AffineConversion=off
  Passive_force_norm : MATLAB Function  TreatAsAtomicUnit=on
  Rigid Transform : sm_lib/Frames and Transforms/Rigid Transform  TranslationMethod=Cartesian  TranslationStandardOffset=0  TranslationStandardOffsetUnits=m  TranslationStandardAxis=+Z  TranslationCartesianOffset=[1 1 -10]  TranslationCartesianOffsetUnits=m  TranslationROffset=0  TranslationROffsetUnits=m  TranslationZOffset=0  TranslationZOffsetUnits=m  TranslationThetaOffset=0  TranslationThetaOffsetUnits=deg  RotationMethod=None  RotationAngleUnits=deg  RotationStandardAxis=+Z  RotationAngle=0.0  RotationArbitraryAxis=[0 0 1]  FollAlignAxisA=+X  BaseAlignAxisA=+Y  FollAlignAxisB=+Y  BaseAlignAxisB=+Z  RotationSequenceAxes=FollowerAxes  RotationSequence=XYX  RotationSequenceAngles=[0 0 0]  RotationSequenceAnglesUnits=deg  RotationMatrix=[1 0 0; 0 1 0; 0 0 1]  Quaternion=[1 0 0 0]
  Rigid Transform1 : sm_lib/Frames and Transforms/Rigid Transform  TranslationMethod=Cartesian  TranslationStandardOffset=0  TranslationStandardOffsetUnits=m  TranslationStandardAxis=+Z  TranslationCartesianOffset=[-10 12 0]  TranslationCartesianOffsetUnits=m  TranslationROffset=0  TranslationROffsetUnits=m  TranslationZOffset=0  TranslationZOffsetUnits=m  TranslationThetaOffset=0  TranslationThetaOffsetUnits=deg  RotationMethod=None  RotationAngleUnits=deg  RotationStandardAxis=+Z  RotationAngle=0.0  RotationArbitraryAxis=[0 0 1]  FollAlignAxisA=+X  BaseAlignAxisA=+Y  FollAlignAxisB=+Y  BaseAlignAxisB=+Z  RotationSequenceAxes=FollowerAxes  RotationSequence=XYX  RotationSequenceAngles=[0 0 0]  RotationSequenceAnglesUnits=deg  RotationMatrix=[1 0 0; 0 1 0; 0 0 1]  Quaternion=[1 0 0 0]
  Scope : Scope
  Simulink-PS Converter : nesl_utility/Simulink-PS Converter  PhysicalDomain=network_engine_domain  SubClassName=ps_input  LeftPortType=input  RightPortType=output  PseudoPeriodic=off  Frequencies=[]  NoiseDistribution=none  NoiseParameters=[]  Unit=1  AffineConversion=off  FilteringAndDerivatives=provide  SimscapeFilterOrder=1  InputFilterTimeConstant=0.001  UdotUserProvided=0
  Sum : Sum  Inputs=|++
  Tlak->Tah : Gain
  Transform Sensor : sm_lib/Frames and Transforms/Transform Sensor  MeasurementFrame=World  RotationSequence=XYX  SenseAngle=off  SenseAxis=off  SenseQ=off  SenseR=off  SenseRotationSequence=off  SenseOmegaX=off  SenseOmegaY=off  SenseOmegaZ=off  SenseQDot=off  SenseRDot=off  SenseRotationSequenceDot=off  SenseAlphaX=off  SenseAlphaY=off  SenseAlphaZ=off  SenseQDDot=off  SenseRDDot=off  SenseX=off  SenseY=off  SenseZ=off  SenseRad=off  SenseAzim=off  SenseDist=on  SenseInc=off  SenseXDot=off  SenseYDot=off  SenseZDot=off  SenseRadDot=off  SenseAzimDot=off  SenseDistDot=off  SenseIncDot=off  SenseXDDot=off  SenseYDDot=off  SenseZDDot=off  SenseRadDDot=off  SenseAzimDDot=off  SenseDistDDot=off  SenseIncDDot=off
  l0m : Constant  Value=l0m(1)
  Th : PMIOPort  Side=Left
  Cl : PMIOPort  Port=2  Side=Left
  wires:
  Aktivace/1 -> Active_factor_norm/3(a)
  l0m/1 -> Passive_force_norm/2(l0), Active_factor_norm/2(l0)
  PS-Simulink Converter/1 -> Passive_force_norm/1(lm), Active_factor_norm/1(lm)
  Tlak->Tah/1 -> Simulink-PS Converter/1, Scope/1
  Active_factor_norm/1(Fa_norm) -> Sum/2
  Passive_force_norm/1(Fp_norm) -> Sum/1
  F0M/1 -> Tlak->Tah/1
  Sum/1 -> F0M/1
  connections:
  Cl/RConn1 -- Rigid Transform/LConn1
  Rigid Transform1/LConn1 -- Th/RConn1
  Transform Sensor/RConn2 -- PS-Simulink Converter/LConn1
  Simulink-PS Converter/RConn1 -- Internal Force/LConn2
  Transform Sensor/RConn1 -- Rigid Transform1/RConn1 -- Internal Force/RConn1
  Transform Sensor/LConn1 -- Rigid Transform/RConn1 -- Internal Force/LConn1

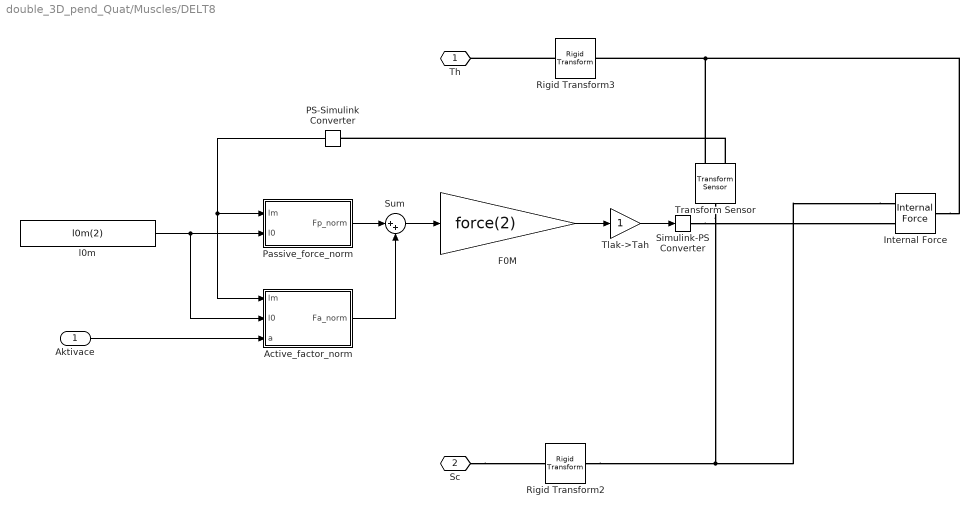
== system double_3D_pend_Quat/Muscles/DELT8 ==
  Aktivace : Inport
  Active_factor_norm : MATLAB Function  TreatAsAtomicUnit=on
  F0M : Gain  Gain=force(2)
  Internal Force : sm_lib/Forces and Torques/Internal Force
  PS-Simulink Converter : nesl_utility/PS-Simulink Converter  PhysicalDomain=network_engine_domain  SubClassName=ps_output  LeftPortType=input  RightPortType=output  PseudoPeriodic=off  Frequencies=[]  VectorFormat=inherit  Unit=inherit  AffineConversion=off
  Passive_force_norm : MATLAB Function  TreatAsAtomicUnit=on
  Rigid Transform2 : sm_lib/Frames and Transforms/Rigid Transform  TranslationMethod=Cartesian  TranslationStandardOffset=0  TranslationStandardOffsetUnits=m  TranslationStandardAxis=+Z  TranslationCartesianOffset=[-1 1 -10]  TranslationCartesianOffsetUnits=m  TranslationROffset=0  TranslationROffsetUnits=m  TranslationZOffset=0  TranslationZOffsetUnits=m  TranslationThetaOffset=0  TranslationThetaOffsetUnits=deg  RotationMethod=None  RotationAngleUnits=deg  RotationStandardAxis=+Z  RotationAngle=0.0  RotationArbitraryAxis=[0 0 1]  FollAlignAxisA=+X  BaseAlignAxisA=+Y  FollAlignAxisB=+Y  BaseAlignAxisB=+Z  RotationSequenceAxes=FollowerAxes  RotationSequence=XYX  RotationSequenceAngles=[0 0 0]  RotationSequenceAnglesUnits=deg  RotationMatrix=[1 0 0; 0 1 0; 0 0 1]  Quaternion=[1 0 0 0]
  Rigid Transform3 : sm_lib/Frames and Transforms/Rigid Transform  TranslationMethod=Cartesian  TranslationStandardOffset=0  TranslationStandardOffsetUnits=m  TranslationStandardAxis=+Z  TranslationCartesianOffset=[-10 12 0]  TranslationCartesianOffsetUnits=m  TranslationROffset=0  TranslationROffsetUnits=m  TranslationZOffset=0  TranslationZOffsetUnits=m  TranslationThetaOffset=0  TranslationThetaOffsetUnits=deg  RotationMethod=None  RotationAngleUnits=deg  RotationStandardAxis=+Z  RotationAngle=0.0  RotationArbitraryAxis=[0 0 1]  FollAlignAxisA=+X  BaseAlignAxisA=+Y  FollAlignAxisB=+Y  BaseAlignAxisB=+Z  RotationSequenceAxes=FollowerAxes  RotationSequence=XYX  RotationSequenceAngles=[0 0 0]  RotationSequenceAnglesUnits=deg  RotationMatrix=[1 0 0; 0 1 0; 0 0 1]  Quaternion=[1 0 0 0]
  Simulink-PS Converter : nesl_utility/Simulink-PS Converter  PhysicalDomain=network_engine_domain  SubClassName=ps_input  LeftPortType=input  RightPortType=output  PseudoPeriodic=off  Frequencies=[]  NoiseDistribution=none  NoiseParameters=[]  Unit=1  AffineConversion=off  FilteringAndDerivatives=provide  SimscapeFilterOrder=1  InputFilterTimeConstant=0.001  UdotUserProvided=0
  Sum : Sum  Inputs=|++
  Tlak->Tah : Gain
  Transform Sensor : sm_lib/Frames and Transforms/Transform Sensor  MeasurementFrame=World  RotationSequence=XYX  SenseAngle=off  SenseAxis=off  SenseQ=off  SenseR=off  SenseRotationSequence=off  SenseOmegaX=off  SenseOmegaY=off  SenseOmegaZ=off  SenseQDot=off  SenseRDot=off  SenseRotationSequenceDot=off  SenseAlphaX=off  SenseAlphaY=off  SenseAlphaZ=off  SenseQDDot=off  SenseRDDot=off  SenseX=off  SenseY=off  SenseZ=off  SenseRad=off  SenseAzim=off  SenseDist=on  SenseInc=off  SenseXDot=off  SenseYDot=off  SenseZDot=off  SenseRadDot=off  SenseAzimDot=off  SenseDistDot=off  SenseIncDot=off  SenseXDDot=off  SenseYDDot=off  SenseZDDot=off  SenseRadDDot=off  SenseAzimDDot=off  SenseDistDDot=off  SenseIncDDot=off
  l0m : Constant  Value=l0m(2)
  Th : PMIOPort  Side=Left
  Sc : PMIOPort  Port=2  Side=Left
  wires:
  Sum/1 -> F0M/1
  F0M/1 -> Tlak->Tah/1
  Passive_force_norm/1(Fp_norm) -> Sum/1
  Active_factor_norm/1(Fa_norm) -> Sum/2
  Tlak->Tah/1 -> Simulink-PS Converter/1
  PS-Simulink Converter/1 -> Active_factor_norm/1(lm), Passive_force_norm/1(lm)
  l0m/1 -> Active_factor_norm/2(l0), Passive_force_norm/2(l0)
  Aktivace/1 -> Active_factor_norm/3(a)
  connections:
  Sc/RConn1 -- Rigid Transform2/LConn1
  Rigid Transform3/LConn1 -- Th/RConn1
  Internal Force/LConn1 -- Rigid Transform2/RConn1 -- Transform Sensor/LConn1
  Internal Force/RConn1 -- Transform Sensor/RConn1 -- Rigid Transform3/RConn1
  Simulink-PS Converter/RConn1 -- Internal Force/LConn2
  Transform Sensor/RConn2 -- PS-Simulink Converter/LConn1

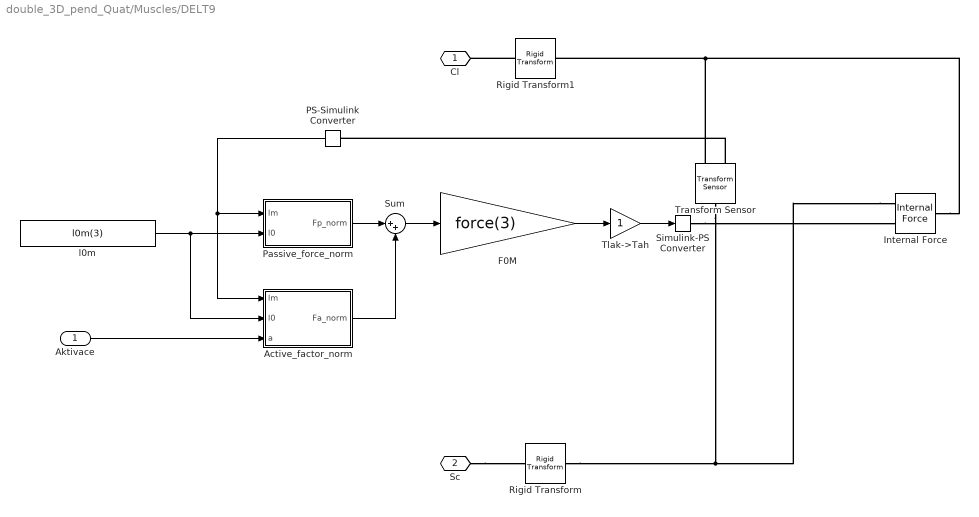
== system double_3D_pend_Quat/Muscles/DELT9 ==
  Aktivace : Inport
  Active_factor_norm : MATLAB Function  TreatAsAtomicUnit=on
  F0M : Gain  Gain=force(3)
  Internal Force : sm_lib/Forces and Torques/Internal Force
  PS-Simulink Converter : nesl_utility/PS-Simulink Converter  PhysicalDomain=network_engine_domain  SubClassName=ps_output  LeftPortType=input  RightPortType=output  PseudoPeriodic=off  Frequencies=[]  VectorFormat=inherit  Unit=inherit  AffineConversion=off
  Passive_force_norm : MATLAB Function  TreatAsAtomicUnit=on
  Rigid Transform : sm_lib/Frames and Transforms/Rigid Transform  TranslationMethod=Cartesian  TranslationStandardOffset=0  TranslationStandardOffsetUnits=m  TranslationStandardAxis=+Z  TranslationCartesianOffset=[1 -6 3]  TranslationCartesianOffsetUnits=m  TranslationROffset=0  TranslationROffsetUnits=m  TranslationZOffset=0  TranslationZOffsetUnits=m  TranslationThetaOffset=0  TranslationThetaOffsetUnits=deg  RotationMethod=None  RotationAngleUnits=deg  RotationStandardAxis=+Z  RotationAngle=0.0  RotationArbitraryAxis=[0 0 1]  FollAlignAxisA=+X  BaseAlignAxisA=+Y  FollAlignAxisB=+Y  BaseAlignAxisB=+Z  RotationSequenceAxes=FollowerAxes  RotationSequence=XYX  RotationSequenceAngles=[0 0 0]  RotationSequenceAnglesUnits=deg  RotationMatrix=[1 0 0; 0 1 0; 0 0 1]  Quaternion=[1 0 0 0]
  Rigid Transform1 : sm_lib/Frames and Transforms/Rigid Transform  TranslationMethod=Cartesian  TranslationStandardOffset=0  TranslationStandardOffsetUnits=m  TranslationStandardAxis=+Z  TranslationCartesianOffset=[-4 5 0]  TranslationCartesianOffsetUnits=m  TranslationROffset=0  TranslationROffsetUnits=m  TranslationZOffset=0  TranslationZOffsetUnits=m  TranslationThetaOffset=0  TranslationThetaOffsetUnits=deg  RotationMethod=None  RotationAngleUnits=deg  RotationStandardAxis=+Z  RotationAngle=0.0  RotationArbitraryAxis=[0 0 1]  FollAlignAxisA=+X  BaseAlignAxisA=+Y  FollAlignAxisB=+Y  BaseAlignAxisB=+Z  RotationSequenceAxes=FollowerAxes  RotationSequence=XYX  RotationSequenceAngles=[0 0 0]  RotationSequenceAnglesUnits=deg  RotationMatrix=[1 0 0; 0 1 0; 0 0 1]  Quaternion=[1 0 0 0]
  Simulink-PS Converter : nesl_utility/Simulink-PS Converter  PhysicalDomain=network_engine_domain  SubClassName=ps_input  LeftPortType=input  RightPortType=output  PseudoPeriodic=off  Frequencies=[]  NoiseDistribution=none  NoiseParameters=[]  Unit=1  AffineConversion=off  FilteringAndDerivatives=provide  SimscapeFilterOrder=1  InputFilterTimeConstant=0.001  UdotUserProvided=0
  Sum : Sum  Inputs=|++
  Tlak->Tah : Gain
  Transform Sensor : sm_lib/Frames and Transforms/Transform Sensor  MeasurementFrame=World  RotationSequence=XYX  SenseAngle=off  SenseAxis=off  SenseQ=off  SenseR=off  SenseRotationSequence=off  SenseOmegaX=off  SenseOmegaY=off  SenseOmegaZ=off  SenseQDot=off  SenseRDot=off  SenseRotationSequenceDot=off  SenseAlphaX=off  SenseAlphaY=off  SenseAlphaZ=off  SenseQDDot=off  SenseRDDot=off  SenseX=off  SenseY=off  SenseZ=off  SenseRad=off  SenseAzim=off  SenseDist=on  SenseInc=off  SenseXDot=off  SenseYDot=off  SenseZDot=off  SenseRadDot=off  SenseAzimDot=off  SenseDistDot=off  SenseIncDot=off  SenseXDDot=off  SenseYDDot=off  SenseZDDot=off  SenseRadDDot=off  SenseAzimDDot=off  SenseDistDDot=off  SenseIncDDot=off
  l0m : Constant  Value=l0m(3)
  Cl : PMIOPort  Side=Left
  Sc : PMIOPort  Port=2  Side=Left
  wires:
  Sum/1 -> F0M/1
  F0M/1 -> Tlak->Tah/1
  Passive_force_norm/1(Fp_norm) -> Sum/1
  Active_factor_norm/1(Fa_norm) -> Sum/2
  Tlak->Tah/1 -> Simulink-PS Converter/1
  PS-Simulink Converter/1 -> Active_factor_norm/1(lm), Passive_force_norm/1(lm)
  l0m/1 -> Active_factor_norm/2(l0), Passive_force_norm/2(l0)
  Aktivace/1 -> Active_factor_norm/3(a)
  connections:
  Internal Force/LConn1 -- Transform Sensor/LConn1 -- Rigid Transform/RConn1
  Internal Force/RConn1 -- Rigid Transform1/RConn1 -- Transform Sensor/RConn1
  Simulink-PS Converter/RConn1 -- Internal Force/LConn2
  Transform Sensor/RConn2 -- PS-Simulink Converter/LConn1
  Rigid Transform1/LConn1 -- Cl/RConn1
  Sc/RConn1 -- Rigid Transform/LConn1

== matlab function double_3D_pend_Quat/Muscles/DELT9/Active_factor_norm ==
  data: Fa_norm output; lm input; l0 input; a input
function Fa_norm = fcn(lm,l0,a)
f_gauss = 0.25;
Fa_norm = (exp(-(lm/l0-1)^2/f_gauss))*a;

== matlab function double_3D_pend_Quat/Muscles/DELT9/Passive_force_norm ==
  data: lm input; Fp_norm output; l0 input
function Fp_norm = fcn(lm,l0)
Fp_norm = ((lm/l0)^3)*exp(8*lm/l0-12.9);

== matlab function double_3D_pend_Quat/MATLAB Function5 ==
  data: u input; Izz parameter; Iyy parameter; Ixx parameter; g parameter; l parameter; m parameter; y output; q1new output; q2new output; akt input; l0m parameter; force parameter
function [y,q1new,q2new]  = fcn(u,Izz, Iyy, Ixx, g, l, m,akt, l0m, force)
t = 0;
% you need to predefine the size of output vector
y = zeros(14,1);

% extract quaternion from the y vector, u(9:11) and u(12:14) are angular
% velocities of joints 1 and 2, respectively
q1 = u(1:4);
q2 = u(5:8);

%renormalize quaternion each step (this is just temporal, It was recommended to me to use for example Gauss-Legendre methods to keep quaternion unit)
q1new = q1/norm(q1);
q2new = q2/norm(q2);

%angular velocities
u1 = u(9:11);
u2 = u(12:end);

FM = FM_quat(0,[q1new;q2new]',force,l0m,akt);
MM = mm_quat(t,[q1new;q2new]',[u1;u2]',Ixx,Iyy,Izz,l,m, g);
FE = fe_quat(t,[q1new;q2new]',[u1;u2]',Ixx,Iyy,Izz,l,m, g);
y = MM\(FE+[zeros(8,1);FM]);
end

== matlab function double_3D_pend_Quat/MATLAB Function6 ==
  data: u input; Izz parameter; Iyy parameter; Ixx parameter; g parameter; l parameter; m parameter; y output; q1new output; q2new output; akt input; l0m parameter; force parameter
function [y,q1new,q2new]  = fcn(u,Izz, Iyy, Ixx, g, l, m,akt, l0m, force)
t = 0;
y = zeros(14,1);
q1 = u(1:4);
q2 = u(5:8);

% the difference here are q1m and q2m, you need to check the first term and
% multiply it by -1 if needed
q1m = u(1:4);
q2m = u(5:8);

if q1(1) < 0
    q1m = q1*-1;
end
%
if q2(1) < 0
    q2m = q2*-1;
end

% normalize both of them
q1newm = q1m/norm(q1m);
q2newm = q2m/norm(q2m);
q1new = q1/norm(q1);
q2new = q2/norm(q2);
u1 = u(9:11);
u2 = u(12:end);

% q1m and q2m goes into the muscle force function
FM = FM_quat_Cnst(0,[q1newm;q2newm]',force,l0m,akt);
MM = mm_quat(t,[q1new;q2new]',[u1;u2]',Ixx,Iyy,Izz,l,m, g);
FE = fe_quat(t,[q1new;q2new]',[u1;u2]',Ixx,Iyy,Izz,l,m, g);
y = MM\(FE+[zeros(8,1);FM]);
end

== matlab function double_3D_pend_Quat/Muscles/DELT10/Active_factor_norm ==
  data: Fa_norm output; lm input; l0 input; a input
function Fa_norm = fcn(lm,l0,a)
f_gauss = 0.25;
Fa_norm = (exp(-(lm/l0-1)^2/f_gauss))*a;

== matlab function double_3D_pend_Quat/Muscles/DELT10/Passive_force_norm ==
  data: lm input; Fp_norm output; l0 input
function Fp_norm = fcn(lm,l0)
Fp_norm = ((lm/l0)^3)*exp(8*lm/l0-12.9);

== matlab function double_3D_pend_Quat/Muscles/DELT11/Active_factor_norm ==
  data: Fa_norm output; lm input; l0 input; a input
function Fa_norm = fcn(lm,l0,a)
f_gauss = 0.25;
Fa_norm = (exp(-(lm/l0-1)^2/f_gauss))*a;

== matlab function double_3D_pend_Quat/Muscles/DELT11/Passive_force_norm ==
  data: lm input; Fp_norm output; l0 input
function Fp_norm = fcn(lm,l0)
Fp_norm = ((lm/l0)^3)*exp(8*lm/l0-12.9);

== matlab function double_3D_pend_Quat/Muscles/DELT12/Active_factor_norm ==
  data: Fa_norm output; lm input; l0 input; a input
function Fa_norm = fcn(lm,l0,a)
f_gauss = 0.25;
Fa_norm = (exp(-(lm/l0-1)^2/f_gauss))*a;

== matlab function double_3D_pend_Quat/Muscles/DELT12/Passive_force_norm ==
  data: lm input; Fp_norm output; l0 input
function Fp_norm = fcn(lm,l0)
Fp_norm = ((lm/l0)^3)*exp(8*lm/l0-12.9);

== matlab function double_3D_pend_Quat/Muscles/DELT7/Active_factor_norm ==
  data: Fa_norm output; lm input; l0 input; a input
function Fa_norm = fcn(lm,l0,a)
f_gauss = 0.25;
Fa_norm = (exp(-(lm/l0-1)^2/f_gauss))*a;

== matlab function double_3D_pend_Quat/Muscles/DELT7/Passive_force_norm ==
  data: lm input; Fp_norm output; l0 input
function Fp_norm = fcn(lm,l0)
Fp_norm = ((lm/l0)^3)*exp(8*lm/l0-12.9);

== matlab function double_3D_pend_Quat/Muscles/DELT8/Active_factor_norm ==
  data: Fa_norm output; lm input; l0 input; a input
function Fa_norm = fcn(lm,l0,a)
f_gauss = 0.25;
Fa_norm = (exp(-(lm/l0-1)^2/f_gauss))*a;

== matlab function double_3D_pend_Quat/Muscles/DELT8/Passive_force_norm ==
  data: lm input; Fp_norm output; l0 input
function Fp_norm = fcn(lm,l0)
Fp_norm = ((lm/l0)^3)*exp(8*lm/l0-12.9);
